simulink model "exp2_3_2_P"  (R2014a)
settings: Solver=ode5  StartTime=0.0  StopTime=inf  RelTol=1e-3
libraries: slrtlib x3, xpcdiamondlib x2
settings Model: BufferReuse=off  Creator=dallen6  LastModifiedBy=dallen6
settings SolverCC: EnableConcurrentExecution=on
settings OptimizationCC: BlockReduction=off  OptimizeBlockIOStorage=off  BufferReuse=off  GlobalBufferReuse=off  ExpressionFolding=off  LocalBlockOutputs=off
settings HardwareCC: ProdIntDivRoundTo=Zero  ProdEndianess=LittleEndian  ProdHWDeviceType=Generic->32-bit x86 compatible
settings RTWCC: SystemTargetFile=slrt.tlc  TemplateMakefile=slrt_default_tmf  Description=Simulink Real-Time  ProcessScript=slrt_make_rtw_hook  RTWCompilerOptimization=On
settings SimulinkRealTimeCC: GeneratePreprocessorConditionals=Disable all  EnableShiftOperators=on

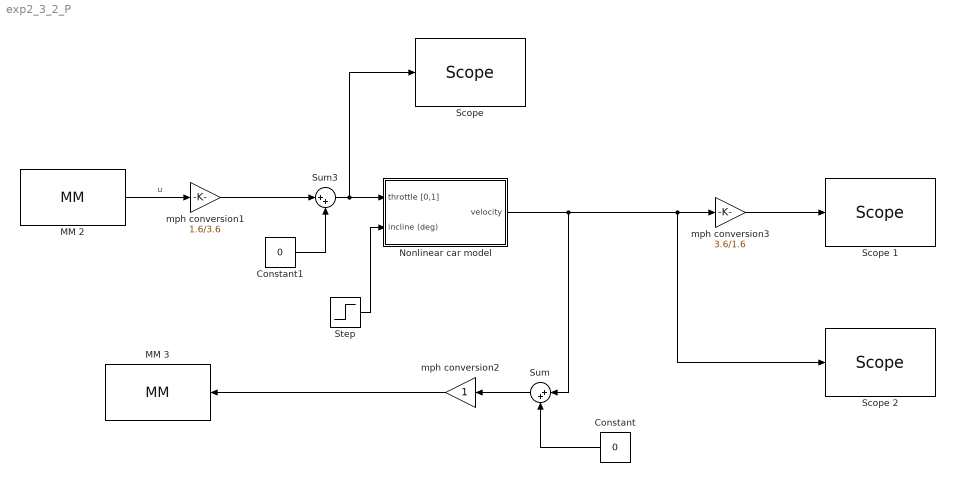
== system exp2_3_2_P ==
  Constant : Constant  Value=0
  Constant1 : Constant  Value=0
  MM 2 : xpcdiamondlib/A//D/MM   numChans=1  range=-5V to 5V  coupling=16 single-ended channels  showStatus=off  sampleTime=0.01  base=0x300
  MM 3 : xpcdiamondlib/D//A/MM   channel=[1]  range=[5]  reset=[1]  initValue=[0]  sampleTime=0.01  base=0x300
  Nonlinear car model : Subsystem  mask{ca=1*1500, cf=1*1500/55/55, m=1500}
      mask prompts: ca "acceleration coeff"; cf "friction/aero coeff"; m "mass"
  "Scope " : slrtlib/Displays and Logging/Scope   scopeno=3  scopetype=File  autostart=on  viewmode=Graphical redraw  formatstr='%15.6f'  grid=on  ylimits=[0,0]  nosamples=5000  noprepostsamples=0  interleave=1  triggermode=FreeRun  triggersignal=1  trigsignalfromport=off  triggerlevel=0.0  triggerslope=Either  triggerscope=1  triggersample=0  filename=datap3.dat  mode=Lazy  writesize=512  autorestart=on  dynamicfilemode=off  maxwritefilesize=512*1024^2
  Scope 1 : slrtlib/Displays and Logging/Scope   scopeno=1  scopetype=File  autostart=on  viewmode=Graphical redraw  formatstr='%15.6f'  grid=on  ylimits=[0,0]  nosamples=5000  noprepostsamples=0  interleave=1  triggermode=FreeRun  triggersignal=1  trigsignalfromport=off  triggerlevel=0.0  triggerslope=Either  triggerscope=1  triggersample=0  filename=datap1.dat  mode=Lazy  writesize=512  autorestart=on  dynamicfilemode=off  maxwritefilesize=512*1024^2
  Scope 2 : slrtlib/Displays and Logging/Scope   scopeno=2  scopetype=File  autostart=on  viewmode=Graphical redraw  formatstr='%15.6f'  grid=on  ylimits=[0,0]  nosamples=5000  noprepostsamples=0  interleave=1  triggermode=FreeRun  triggersignal=1  trigsignalfromport=off  triggerlevel=0.0  triggerslope=Either  triggerscope=1  triggersample=0  filename=datap2.dat  mode=Lazy  writesize=512  autorestart=on  dynamicfilemode=off  maxwritefilesize=512*1024^2
  Step : Step  Time=10  Before=60  After=65  SampleTime=0
  Sum : Sum  Inputs=|++
  Sum3 : Sum  Inputs=|++
  mph conversion1 : Gain  Gain=1.6/3.6  SaturateOnIntegerOverflow=on  OutDataTypeStr=Inherit: Same as input  ParamDataTypeStr=Inherit: Same as input
  mph conversion2 : Gain  SaturateOnIntegerOverflow=on  OutDataTypeStr=Inherit: Same as input  ParamDataTypeStr=Inherit: Same as input
  mph conversion3 : Gain  Gain=3.6/1.6  SaturateOnIntegerOverflow=on  OutDataTypeStr=Inherit: Same as input  ParamDataTypeStr=Inherit: Same as input
  wires:
  MM 2/1 -> mph conversion1/1  "u"
  mph conversion1/1 -> Sum3/1
  Constant1/1 -> Sum3/2
  Sum3/1 -> "Scope "/1, Nonlinear car model/1(throttle [0,1])
  mph conversion2/1 -> MM 3/1
  Sum/1 -> mph conversion2/1
  Constant/1 -> Sum/2
  Step/1 -> Nonlinear car model/2(incline (deg))
  Nonlinear car model/1(velocity) -> Sum/1, Scope 2/1, mph conversion3/1
  mph conversion3/1 -> Scope 1/1

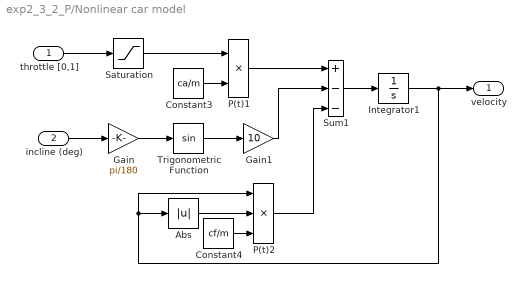
== system exp2_3_2_P/Nonlinear car model ==
  throttle [0,1] : Inport
  incline (deg) : Inport  Port=2
  Abs : Abs  SaturateOnIntegerOverflow=on
  Constant3 : Constant  Value=ca/m
  Constant4 : Constant  Value=cf/m
  Gain : Gain  Gain=pi/180  SaturateOnIntegerOverflow=on  OutDataTypeStr=Inherit: Same as input  ParamDataTypeStr=Inherit: Same as input
  Gain1 : Gain  Gain=10  SaturateOnIntegerOverflow=on  OutDataTypeStr=Inherit: Same as input  ParamDataTypeStr=Inherit: Same as input
  Integrator1 : Integrator  InitialCondition=26.67  UpperSaturationLimit=1  LowerSaturationLimit=0
  P(t)1 : Product  Inputs=**  SaturateOnIntegerOverflow=on  RndMeth=Zero  InputSameDT=on  OutDataTypeStr=Inherit: Same as first input
  P(t)2 : Product  Inputs=***  SaturateOnIntegerOverflow=on  RndMeth=Zero  InputSameDT=on  OutDataTypeStr=Inherit: Same as first input
  Saturation : Saturate  UpperLimit=3  LowerLimit=-1
  Sum1 : Sum  Inputs=+--  SaturateOnIntegerOverflow=on  InputSameDT=on  OutDataTypeStr=Inherit: Same as first input
  Trigonometric Function : Trigonometry
  velocity : Outport
  wires:
  Saturation/1 -> P(t)1/1
  Sum1/1 -> Integrator1/1
  Constant3/1 -> P(t)1/2
  P(t)1/1 -> Sum1/1
  Integrator1/1 -> Abs/1, P(t)2/1, velocity/1
  Constant4/1 -> P(t)2/3
  throttle [0,1]/1 -> Saturation/1
  incline (deg)/1 -> Gain/1
  P(t)2/1 -> Sum1/3
  Gain/1 -> Trigonometric Function/1
  Gain1/1 -> Sum1/2
  Trigonometric Function/1 -> Gain1/1
  Abs/1 -> P(t)2/2
